simulink model "HVDC_VSC_1CPUcore_dcpl"  (Simulink 8.4)
settings: Solver=ode3  SolverMode=SingleTasking  StartTime=0.0  StopTime=70.0  FixedStep=Ts_Power  RelTol=1e-3  AbsTol=1e-2
PreLoadFcn:
  | Ts_Power=50e-6; Ts_Control=1*Ts_Power; init_cosim_IA; startup_transients_hvdc_vsc;
PostLoadFcn:
  | Ts_Power=50e-6; Ts_Control=1*Ts_Power; init_cosim_IA; startup_transients_hvdc_vsc;
InitFcn:
  | Ts_Power=50e-6; Ts_Control=1*Ts_Power; init_cosim_IA; startup_transients_hvdc_vsc;
values from neighbouring files (symbols this model uses):
  dPref1_2 = 0.125    [startup_transients_hvdc_vsc.m]
  dPref1_2_rlimit = 0.6    [startup_transients_hvdc_vsc.m]
  t_deblock_Pref1 = 0.5    [startup_transients_hvdc_vsc.m]
  t_deblock_Udref2 = 0.3    [startup_transients_hvdc_vsc.m]
  t_dPref1_2 = 25.0    (= 25)    [startup_transients_hvdc_vsc.m]
  t_SwitchITMIdc = 0.2    [startup_transients_hvdc_vsc.m]
  t_SwitchITMVdc = 0.1    [startup_transients_hvdc_vsc.m]
undefined symbols (not defined in the file or in its folder): CLARK, D1, Delta, gcbh, h, intfDelay, level, lib_mesures, magnitude, ResistanceM, rte_drive_private_lib, rte_tsb3level_hiz_rect_cb, sps_rtmsupport, Ts_intf, TSB3_hiZR
libraries: powerlib x183, spsVIMeasurementModel x102, powerlib_extras x71, powerlib_meascontrol x50, rteventslib x26, op_dpl_lib x20, rtlab x12, sps_avr x6, artemis x1
(part 3 of 13)

== system HVDC_VSC_1CPUcore_dcpl/SM_HVDC_VSC/VSC Controller (Station 2) ==
  note: VSC Controller
      | (Station 2)
  note: |----------------Ts_Power--------------|
  note: Sample time:
  note: |------------Ts_Power------------|
  note: |---------------------------Ts_Control-------------------------|
  note: Reference Steps
  note: RTE Firing Pulse unit
  2*pi1 : Gain  Gain=2*pi  SaturateOnIntegerOverflow=on  OutDataTypeStr=Inherit: Same as input  ParamDataTypeStr=Inherit: Same as input
  3-level firing pulse unit for TSB : Subsystem  mask(3-phase RT-Event Discrete PWM Generator){Ts=Ts_Power}
      mask prompts: Ts "Sample time:"
  Anti-aliasing Filters : Subsystem  mask(Anti-aliasing (2nd order lowpass)){f0_aa=2000, Ts=Ts_Power}
      mask prompts: f0_aa "Cut-off frequency (Hz):"; Ts "Sample time:"
      mask init:
      | zeta = 1/sqrt(2);
  Block : Step  Time=t_deblock_Udref2  Before=1  After=0  SampleTime=Ts_Control
  Constant{1..3,5..6} (5 alike) : Constant  Value=0
  Constant4 : Constant  Value=0.0
  Constant7 : Constant  Value=0.0
  Constant8 : Constant  Value=1.0
  Discrete 3-phase PWM Generator : powerlib_extras/Discrete  Control Blocks/Discrete 3-phase PWM Generator  ModulatorType=3-level  ModulatorMode=Un-synchronized  nF=27  Fc=27*60  ModulatingSignals=off  m=0.86  Freq=50  Phase=-50  Ts=Ts_Power
  Discrete VSC Controller (Station 2) : Subsystem  mask(Discrete VSC-Based HVDC Controller){Mode=DC Voltage & Reactive  Power, Xnom=[230e3, 100e3, 200e3, 200e6], XP=[20.0, 1.0, -1.0, 1.43], Xdvco=[3.0, 3.0, 1.05, 0.9], XUdc=[2.0, 40.0 ], XQ=[20.0, 0.5, -0.5], Xvco=[3.0, 3.0, 1.05, 0.94], Xcrc=[1.1,  0.8], Xaccc=[0.6, 6.0,  0.3], enable_dcvbc=on, Xdcvbc=[0.2, 0.03], Ts_Control=Ts_Control}
      mask prompts: Mode "Control Mode:"; Xnom "Nominal Voltages and Power: [ Vpcc(Vrms L-L) , Vconv (Vrms L-L),  Vdc (V L-L), Pnom (VA) ]"; XP "P Regulator [ Ki (1/s), Pmax (pu), Pmin (pu), Ramp (pu/s)]"; Xdvco "P Control: Udc Override [ Kp, Ki (1/s), Udc_max (pu), Udc_min (pu)]"; XUdc "DC Voltage Regulator [ Kp, Ki (1/s)]"; XQ "Q Regulator [ Ki (1/s), Qmax (pu), Qmin (pu)]"; Xvco "Q Control: Uac Override [ Kp, Ki (1/s), U_max (pu), U_min (pu)]"; Xcrc "Current Reference Limits [ lim_d (pu),  lim_q (pu)]"; Xaccc "Inner Current Regulator [ Kp, Ki (1/s), Kf (pu)]"; enable_dcvbc "DC Voltage Balance"; Xdcvbc "DC Voltage Balance Control} [ Kp, Ki (1/s)]"; Ts_Control "Sample Time (s)"
      mask help:
      | This block implements a controller for a VSC (Voltage-Sourced Converter) HVDC using a three-level or Neutral Point Clamped (NPC) converter bridge.
      | The 'Vref_abc' output contains the three modulating signals used by  the carrier-based  Sinusoidal Pulse Width Modulation (SPWM) pulse generator.
      | The output  'm' is a bus signal . Use the Bus Selector block to extract individual signals.
      |
      | See the "VSC-Based Transmission Link " tutorial for a description of the control system.
      mask init: same as HVDC_VSC_1CPUcore_dcpl/SM_HVDC_VSC/VSC Controller (Station 1)/Discrete VSC Controller (Station 1)
      mask TypeOptions Mode: Active & Reactive Power | DC Voltage & Reactive  Power
      mask Callback Mode:
      | tempMaskVis=get_param(gcb,'MaskVisibilities');
      | if strcmp(get_param(gcb,'Mode'),'Active & Reactive Power')
      | 	tempMaskVis{2}='on'; tempMaskVis{3}='on'; tempMaskVis{4}='on'; tempMaskVis{5}='on';
      | 	tempMaskVis{6}='on'; tempMaskVis{5}='off'; tempMaskVis{8}='on'; tempMaskVis{9}='on';
      | 	tempMaskVis{10}='on';  tempMaskVis{12}='on';
      | 
      | else
      | 	tempMaskVis{2}='on'; tempMaskVis{3}='off'; tempMaskVis{4}='off'; tempMaskVis{5}='on';
      | 	tempMaskVis{6}='on'; tempMaskVis{7}='on'; tempMaskVis{8}='on'; tempMaskVis{9}='on';
      | 	tempMaskVis{10}='on';  tempMaskVis{12}='on';
      | end
      | if strcmp(get_param(gcb,'enable_dcvbc'),'on')
      | 	tempMaskVis{11}='on';
      | else
      | 	tempMaskVis{11}='off';
      | end
      | set_param(gcb,'MaskVisibilities',tempMaskVis);
      mask Callback enable_dcvbc:
      | tempMaskVis=get_param(gcb,'MaskVisibilities');
      | if strcmp(get_param(gcb,'enable_dcvbc'),'on')
      | 	tempMaskVis{11}='on';
      | else
      | 	tempMaskVis{11}='off';
      | end
      | set_param(gcb,'MaskVisibilities',tempMaskVis);
  Discrete-Time Integrator2 : DiscreteIntegrator  SampleTime=Ts_Power
  Sum3 : Sum  SaturateOnIntegerOverflow=on
  Switch : Switch  Threshold=0.5  SaturateOnIntegerOverflow=on
  Switch1 : Switch  Threshold=0.5  SaturateOnIntegerOverflow=on
  Switch2 : Switch  Threshold=0.5  SaturateOnIntegerOverflow=on
  Switching_Frequency : Constant  Value=27*60
  Terminator : Terminator
  Unit Delay : UnitDelay  SampleTime=Ts_Control
  tag scope: Control2=global, Pulses2=global, Qref2=global, Udref2=global, Vref_abc2=global
  wires:
  Block/1 -> Switch/2, Discrete VSC Controller (Station 2)/11(block_status), Switch1/2
  Discrete 3-phase PWM Generator/1 -> Switch/3
  Constant2/1 -> Switch/1
  Unit Delay/1 -> Discrete 3-phase PWM Generator/1, 3-level firing pulse unit for TSB/1(3 phase output frequency)
  [Iv_abc2] -> Anti-aliasing Filters/4("Iv_abc ")
  [Uf_abc2] -> Anti-aliasing Filters/3("Uf_abc  ")
  [Iabc_B2] -> Anti-aliasing Filters/2("Iabc ")
  [Uabc_B2] -> Anti-aliasing Filters/1("Uabc ")
  Discrete 3-phase PWM Generator/2 -> Terminator/1
  [VdcPN2] -> Anti-aliasing Filters/5("Udc_pn  ")
  [IdcPN2] -> Anti-aliasing Filters/6("Idc_pn ")
  Anti-aliasing Filters/1(Uabc) -> Discrete VSC Controller (Station 2)/1(Uabc (pu))
  Anti-aliasing Filters/2(Iabc) -> Discrete VSC Controller (Station 2)/2(Iabc (pu))
  Anti-aliasing Filters/3(Uf_abc) -> Discrete VSC Controller (Station 2)/3(Uf_abc (pu))
  Anti-aliasing Filters/4(" Iv_abc") -> Discrete VSC Controller (Station 2)/4(Iv_abc (pu))
  Anti-aliasing Filters/5("Udc_pn ") -> Discrete VSC Controller (Station 2)/5(Udc_pn (pu))
  Anti-aliasing Filters/6(" Idc_pn") -> Discrete VSC Controller (Station 2)/6(Idc_pn (pu))
  Constant3/1 -> Discrete VSC Controller (Station 2)/7(Pref)
  Constant8/1 -> [Udref2], Discrete VSC Controller (Station 2)/10(Udref)
  Constant1/1 -> Discrete VSC Controller (Station 2)/8(dPref)
  Discrete VSC Controller (Station 2)/2(m) -> [Control2]
  Discrete VSC Controller (Station 2)/1(Vref_abc) -> Unit Delay/1, [Vref_abc2]
  3-level firing pulse unit for TSB/1(duty) -> Switch1/3
  Constant5/1 -> Switch1/1
  Discrete-Time Integrator2/1 -> 3-level firing pulse unit for TSB/2(wt)
  2*pi1/1 -> Discrete-Time Integrator2/1
  Switching_Frequency/1 -> 2*pi1/1
  Switch1/1 -> Switch2/3
  Switch/1 -> Switch2/1
  Switch2/1 -> [Pulses2]
  Constant6/1 -> Switch2/2
  Constant4/1 -> Sum3/1
  Sum3/1 -> [Qref2], Discrete VSC Controller (Station 2)/9(Qref)
  Constant7/1 -> Sum3/2
